simulink model "discretetime"  (R2014a)
settings: Solver=ode1  StartTime=0.0  StopTime=15  FixedStep=0.012  MaxStep=0.01  RelTol=0.001
settings Model: SimulationMode=rapid-accelerator  ExtModeTrigDuration=100  Creator=pc  LastModifiedBy=YY
settings SolverCC: MaxConsecutiveZCs=10000
settings DataIOCC: SaveFinalState=on  SaveFormat=StructureWithTime  SaveOutput=off  SaveState=on  StateSaveName=tmp_raccel_xout  SignalLoggingName=tmp_raccel_logsout
settings OptimizationCC: EfficientMapNaN2IntZero=off
settings DebuggingCC: MergeDetectMultiDrivingBlocksExec=error  FrameProcessingCompatibilityMsg=error
settings HardwareCC: TargetLongLongMode=on  TargetIntDivRoundTo=Zero  TargetEndianess=LittleEndian  TargetHWDeviceType=MATLAB Host  ProdEqTarget=off
settings RTWCC: SystemTargetFile=raccel.tlc  TemplateMakefile=raccel_default_tmf  RTWVerbose=off  ProcessScript=raccel_make_rtw_hook  RTWUseSimCustomCode=on
settings CodeAppCC: GenerateComments=off  MaxIdLength=128  SimulinkBlockComments=off
settings RaccelTargetCC: ERTMultiwordTypeDef=System defined  ERTMultiwordLength=256  GeneratePreprocessorConditionals=Disable all  ERTFirstTimeCompliant=off  MultiInstanceERTCode=off  EnableShiftOperators=on  ExtModeMexArgs='', 0, 51334  ENABLE_SLEXEC_SSBRIDGE=0  RTWCAPIParams=off

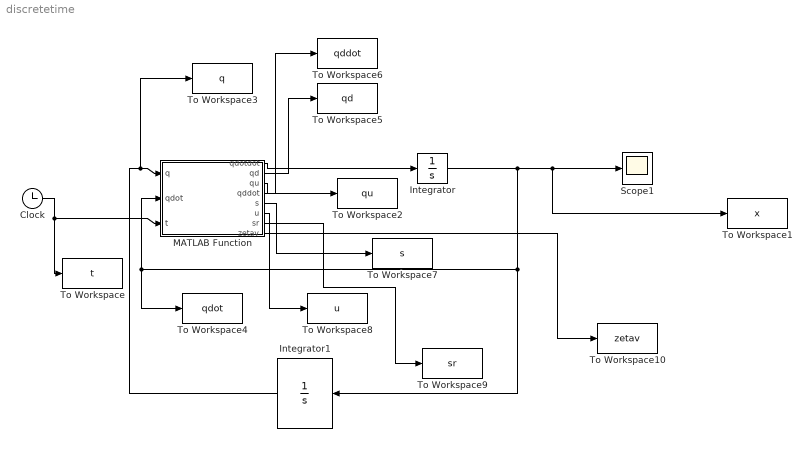
== system discretetime ==
  Clock : Clock
  Integrator : Integrator  InitialCondition=[0;0]
  Integrator1 : Integrator  InitialCondition=[1;0.8]
  MATLAB Function : MATLAB Function  TreatAsAtomicUnit=on
  Scope1 : Scope
      settings: TimeRange=20  YMin=-0.30549  YMax=0.3034
  To Workspace : ToWorkspace  VariableName=t  SampleTime=-1
  To Workspace1 : ToWorkspace  VariableName=x  SampleTime=-1
  To Workspace10 : ToWorkspace  VariableName=zetav  SampleTime=-1
  To Workspace2 : ToWorkspace  VariableName=qu  SampleTime=-1
  To Workspace3 : ToWorkspace  VariableName=q  SampleTime=-1
  To Workspace4 : ToWorkspace  VariableName=qdot  SampleTime=-1
  To Workspace5 : ToWorkspace  VariableName=qd  SampleTime=-1
  To Workspace6 : ToWorkspace  VariableName=qddot  SampleTime=-1
  To Workspace7 : ToWorkspace  VariableName=s  SampleTime=-1
  To Workspace8 : ToWorkspace  VariableName=u  SampleTime=-1
  To Workspace9 : ToWorkspace  VariableName=sr  SampleTime=-1
  wires:
  Integrator/1 -> MATLAB Function/2(qdot), To Workspace4/1, Integrator1/1, To Workspace1/1, Scope1/1
  Clock/1 -> To Workspace/1, MATLAB Function/3(t)
  Integrator1/1 -> To Workspace3/1, MATLAB Function/1(q)
  MATLAB Function/1(qdotdot) -> Integrator/1
  MATLAB Function/2(qd) -> To Workspace5/1
  MATLAB Function/4(qddot) -> To Workspace6/1
  MATLAB Function/5(s) -> To Workspace7/1
  MATLAB Function/3(qu) -> To Workspace2/1
  MATLAB Function/7(sr) -> To Workspace9/1
  MATLAB Function/6(u) -> To Workspace8/1
  MATLAB Function/8(zetav) -> To Workspace10/1

== matlab function discretetime/MATLAB Function ==
  data: qdotdot output; q input; qdot input; t input; qd output; qu output; qddot output; s output; u output; sr output; zetav output

function [qdotdot,qd,qu,qddot,s,u,sr,zetav] = fcn(q,qdot,t)

  miu=0.02;

       miu1=0.02;     
epsilon=0.2;

J1=5;
J2=5;
r1=1;
r2=0.8;
m1=0.5;
m2=1.5;

ld=3;
lf=15;
lq=0.23;

c1=0.4;
C=[c1 0 c1 0; 0 1 0 1];



lm=8.92;
lM=12.52;
gamma=lm/lM;


qd=[0.1*sin(t/3) 0.2*sin(2.5*t)]';
qddot=[0.1/3*cos(t/3) 0.5*cos(2.5*t)]';
qddot2=[-0.1/9*sin(t/3) -1.75*sin(2.5*t)]';

d = [2*sin(t)+rand()-0.5 cos(2*t)+rand()-0.5 ]'; 
q1=q(1);
q2=q(2);
M0 =[(m1+m2)*r1^2+m2*r2^2+J1+2*m2*r1*r2*cos(q2) m2*r2^2+m2*r1*r2*cos(q2); m2*r2^2+m2*r1*r2*cos(q2) m2*r2^2+J2];

b12 = m2*r1*r2*sin(q(2));
dq1=qdot(1);
dq2=qdot(2);
C0 = b12*[-dq1 -2*dq1; 0 dq2];
G0=9.8*[(m1+m2)*r1*cos(q2)+m2*r2*cos(q1+q2);m2*r2*cos(q1+q2)];
f0=-inv(M0)*(C0*qdot+G0);

quaq=miu*round(q/miu);
quaqdot=miu*round(qdot/miu);
zeta1 = quaq-qd;
zeta2 = quaqdot-qddot;


zetav=[q-qd; qdot-qddot];

zeta = [zeta1; zeta2;qd; qddot; qddot2];

sr=C*zeta(1:4);

  qdtrigger =zeta(5:6);  
  
  q2g=zeta(2)+qdtrigger(2);
     q1g=zeta(1)+qdtrigger(1);
  
     qddottrigger =zeta(7:8);
       qddotdottrigger  =zeta(9:10);
   qdot1g = zeta(3)+qddottrigger(1);
   qdot2g = zeta(4)+qddottrigger(2);

  

   
 qg = [q1g;q2g];
   
qdotg = [qdot1g;qdot2g];

b12t = m2*r1*r2*sin(q2g);
dq1g = qdotg(1);
dq2g = qdotg(2);


Mt = [(m1+m2)*r1^2+m2*r2^2+J1+2*m2*r1*r2*cos(q2g) m2*r2^2+m2*r1*r2*cos(q2g); m2*r2^2+m2*r1*r2*cos(q2g) m2*r2^2+J2];

Ct = b12t*[-dq1g -2*dq1g; 0 dq2g];
Gt = 9.8*[(m1+m2)*r1*cos(q2g)+m2*r2*cos(q1g+q2g);m2*r2*cos(q1g+q2g)];
ft = -inv(Mt)*(Ct*qdotg+Gt);

   s      = C*zeta(1:4);
   zeta2g = [zeta(3:4)];

alafa=(1/gamma)*(0.5*sqrt(2)*(miu1/lm+miu*(c1+sqrt(2)*lf))+ld/lm+lq*(1-gamma)+(1-gamma)*(c1*norm(zeta2g)+norm(ft)))+0.1;
    if abs(s(1))>epsilon
      sat1=sign(s(1));
    else
       sat1=s(1)/epsilon;
    end
    
     if abs(s(2))>epsilon
      sat2=sign(s(2));
    else
       sat2=s(2)/epsilon;
    end
    satt=[sat1;sat2];
    
  satt=[sign(s(1));sign(s(2))];
   u=-Mt*(ft- qddotdottrigger +c1*zeta2g + alafa*satt);    

 qu = miu1*round(u/miu1);

qdotdot = f0+inv(M0)*( qu + d);
